simulink model "random_scenario"  (R2025b)
settings: Solver=VariableStepAuto  StartTime=0.0  StopTime=10.0  RelTol=1e-3
undefined symbols (not defined in the file): entity, m, n
settings Model: Creator=39389  LastModifiedBy=39389

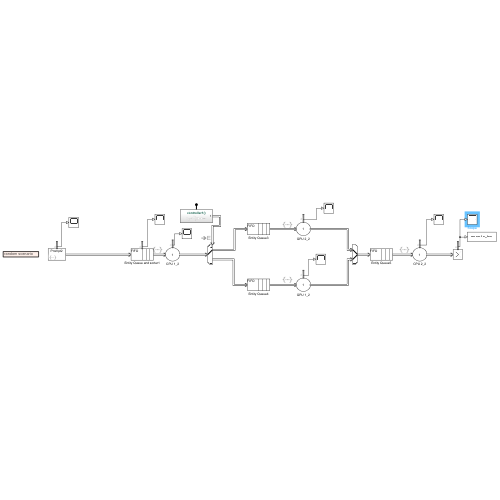
[thumbnail: Simulink's stored preview of the top-level diagram]
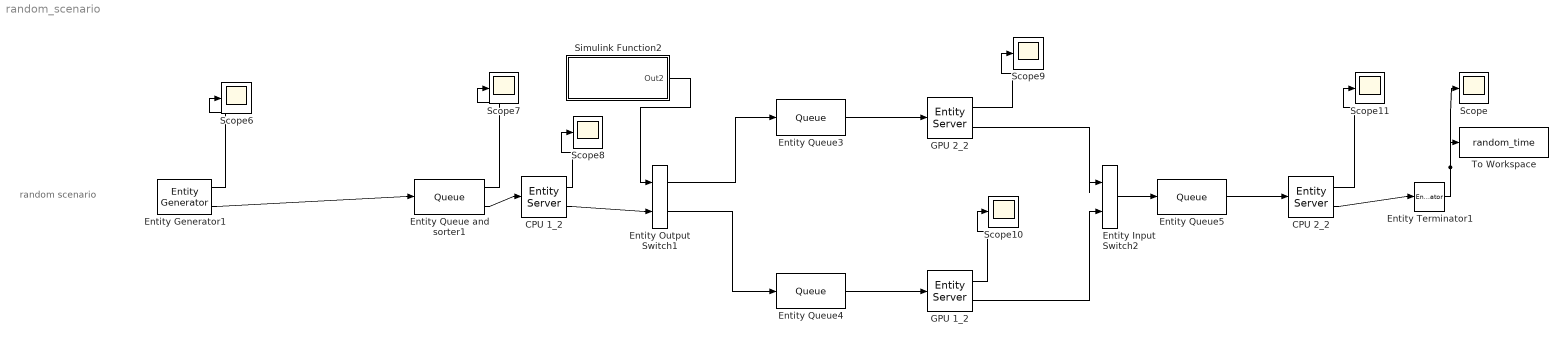
== system random_scenario ==
  note: random scenario
  CPU 1_2 : EntityServer  InputPortMessageModes=m  OutputPortMessageModes=n,m  Capacity=1  ServiceTimeSource=Attribute  ServiceTimeValue=CPU  ServiceTimeAttributeName=CPU1_1  EntryAction=%disp(entity.CPU1)  NumberEntitiesDeparted=on
      settings: OutputPortMap=o0,o9
  CPU 2_2 : EntityServer  InputPortMessageModes=m  OutputPortMessageModes=n,m  Capacity=1  ServiceTimeSource=Attribute  ServiceTimeValue=CPU  ServiceTimeAttributeName=CPU2_1  EntryAction=%disp(entity.CPU1)  NumberEntitiesDeparted=on
      settings: OutputPortMap=o0,o9
  Entity Input Switch2 : EntityInputSwitch  InputPortMessageModes=m,m  OutputPortMessageModes=m
  Entity Output Switch1 : EntityOutputSwitch  InputPortMessageModes=m,m  OutputPortMessageModes=m,m  SwitchingCriterion=From control port  SwitchAttributeName=X
      settings: InputPortMap=u0,u1
  Entity Generator1 : EntityGenerator  OutputPortMessageModes=n,m  TimeSource=MATLAB action  IntergenerationTimeAction=|  GenerateAction=|  AttributeName=ID_1|CPU1_1|X_1|GPU1_1|GPU2_1|CPU2_1|priority_1  AttributeInitialValue=1|0|0|0|0|0|0  NumberEntitiesDeparted=on  EntityType=Structured  EntityTypeName=Prompt2
      IntergenerationTimeAction=|
      | persistent idx itg;
      | 
      | itg = [zeros(1, N), Inf];
      | 
      | if(isempty(idx))
      |     idx = 1;
      |     dt = itg(idx);
      |     idx = idx + 1;
      | end
      | 
      | dt = itg(idx);
      | idx = idx + 1;
      GenerateAction=|
      | entity.ID_1=mod(entitySys.id,Np+1);
      | entity.CPU1_1=P(1,entity.ID_1);
      | entity.GPU1_1=P(2,entity.ID_1);
      | entity.GPU2_1=P(3,entity.ID_1);
      | entity.CPU2_1=P(4,entity.ID_1);
      | %entity.X_1=x_opt(entity.ID_1)+1;
      settings: OutputPortMap=o0,o3
  Entity Queue and sorter1 : Queue  InputPortMessageModes=m  OutputPortMessageModes=n,m  PrioritySource=priority  NumberEntitiesDeparted=on
      settings: OutputPortMap=o0,o5
  Entity Queue3 : Queue  InputPortMessageModes=m  OutputPortMessageModes=m
  Entity Queue4 : Queue  InputPortMessageModes=m  OutputPortMessageModes=m
  Entity Queue5 : Queue  InputPortMessageModes=m  OutputPortMessageModes=m
  Entity Terminator1 : EntityTerminator  InputPortMessageModes=m  NumberEntitiesArrived=on
      settings: OutputPortMap=o0
  GPU 1_2 : EntityServer  InputPortMessageModes=m  OutputPortMessageModes=n,m  Capacity=1  ServiceTimeSource=Attribute  ServiceTimeValue=CPU  ServiceTimeAttributeName=GPU1_1  EntryAction=%disp(entity.CPU1)  NumberEntitiesDeparted=on
      settings: OutputPortMap=o0,o9
  GPU 2_2 : EntityServer  InputPortMessageModes=m  OutputPortMessageModes=n,m  Capacity=1  ServiceTimeSource=Attribute  ServiceTimeValue=CPU  ServiceTimeAttributeName=GPU2_1  EntryAction=%disp(entity.CPU1)  NumberEntitiesDeparted=on
      settings: OutputPortMap=o0,o9
  Scope{,6..11} (7 alike) : Scope
      Scope settings: ActiveDisplayYMinimum=0.43281758957654715  ActiveDisplayYMaximum=5.6828175895765476
      Scope10 settings: ActiveDisplayYMinimum=0.875  ActiveDisplayYMaximum=2.125  DataLoggingVariableName=ScopeData9
      Scope11 settings: ActiveDisplayYMinimum=-1  ActiveDisplayYMaximum=1  DataLoggingVariableName=ScopeData11
      Scope6 settings: ActiveDisplayYMinimum=-1  ActiveDisplayYMaximum=1  DataLoggingVariableName=ScopeData6
      Scope7 settings: ActiveDisplayYMinimum=-1  ActiveDisplayYMaximum=1  DataLoggingVariableName=ScopeData7
      Scope8 settings: ActiveDisplayYMinimum=-1  ActiveDisplayYMaximum=1  DataLoggingVariableName=ScopeData8
      Scope9 settings: DataLoggingVariableName=ScopeData10
  Simulink Function2 : Subsystem  TreatAsAtomicUnit=on
  To Workspace : ToWorkspace  VariableName=random_time  SaveFormat=Timeseries  SampleTime=-1
  wires:
  Entity Output Switch1/1 -> Entity Queue3/1
  CPU 1_2/2 -> Entity Output Switch1/2
  Entity Queue and sorter1/1 -> Scope7/1
  GPU 1_2/2 -> Entity Input Switch2/2
  GPU 2_2/2 -> Entity Input Switch2/1
  Entity Queue4/1 -> GPU 1_2/1
  GPU 1_2/1 -> Scope10/1
  Entity Queue3/1 -> GPU 2_2/1
  CPU 2_2/1 -> Scope11/1
  Entity Generator1/1 -> Scope6/1
  Entity Output Switch1/2 -> Entity Queue4/1
  Entity Queue5/1 -> CPU 2_2/1
  Simulink Function2/1(Out2) -> Entity Output Switch1/1
  GPU 2_2/1 -> Scope9/1
  CPU 1_2/1 -> Scope8/1
  Entity Queue and sorter1/2 -> CPU 1_2/1
  CPU 2_2/2 -> Entity Terminator1/1
  Entity Generator1/2 -> Entity Queue and sorter1/1
  Entity Input Switch2/1 -> Entity Queue5/1
  Entity Terminator1/1 -> To Workspace/1, Scope/1

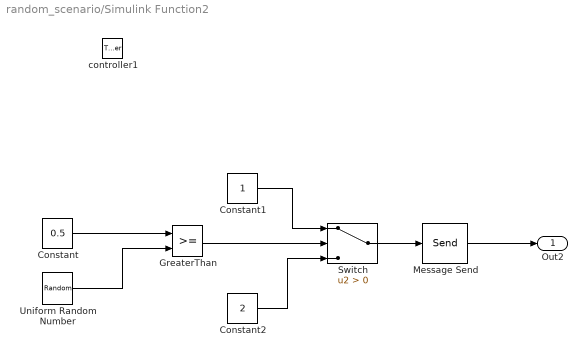
== system random_scenario/Simulink Function2 ==
  controller1 : TriggerPort  TriggerType=function-call  IsSimulinkFunction=on  FunctionName=controller1  FunctionVisibility=scoped  VariantControl=(inherit)
  Constant : Constant  Value=0.5  SampleTime=-1
  Constant1 : Constant
  Constant2 : Constant  Value=2
  GreaterThan : RelationalOperator  OutDataTypeStr=boolean  RndMeth=Simplest  InputSameDT=off
  Message Send : Send  OutputPortMessageModes=m
  Switch : Switch  Criteria=u2 > Threshold  SaturateOnIntegerOverflow=off  InputSameDT=off
  Uniform Random Number : UniformRandomNumber  Minimum=0  Seed=randi(3750)
  Out2 : Outport
  wires:
  GreaterThan/1 -> Switch/2
  Constant1/1 -> Switch/1
  Constant2/1 -> Switch/3
  Switch/1 -> Message Send/1
  Constant/1 -> GreaterThan/1
  Uniform Random Number/1 -> GreaterThan/2
  Message Send/1 -> Out2/1
